simulink model "chydrbf_bruite_s"  (R2017b)
settings: Solver=ode45  StartTime=0.0  StopTime=50  MaxStep=1  MinStep=0.0001  RelTol=1e-8  AbsTol=1e-8  EnableMultiTasking=on
values from neighbouring files (symbols this model uses):
  F = [1 4.73333333333 7.10666666667 8.97333333333 2.88 0.266666666667]    [datahydr_pprTf5.mat]    (also in ppfil.m = real(poly(diag(r))))
  kw = 0.5    [datahydr_pprTf5.mat]    (also in initchydr_yuwch.m)
  R = []    [bezout.m]    (also in datahydr_pprTf5.mat = [1.68 7.4 9.48 11.84 0.8])
  S = []    [bezout.m]    (also in datahydr_pprTf5.mat = [1 4.4 8.64 8.4 5.76 0])
  T = [3 14.2 21.32 26.92 8.64 0.8]    [datahydr_pprTf5.mat]
  Ta = 10    [datahydr_pprTf5.mat]    (also in initchydr_yuwch.m)
  TI = 0.3    [datahydr_pprTf5.mat]    (also in initchydr_yuwch.m)
  Tw = 1    [datahydr_pprTf5.mat]    (also in initchydr_yuwch.m)
settings Model: Creator=pchevrel  LastModifiedBy=pchevrel
settings DataIOCC: LimitDataPoints=on  SaveFormat=Array  SignalLoggingSaveFormat=ModelDataLogs  SaveOutput=off  SaveTime=off  SignalLoggingName=sigsOut
settings OptimizationCC: ExpressionDepthLimit=2147483647  InitFltsAndDblsToZero=on  LifeSpan=inf
settings DebuggingCC: SaveWithParameterizedLinksMsg=none  UnderspecifiedInitializationDetection=Classic  MergeDetectMultiDrivingBlocksExec=none  SignalResolutionControl=TryResolveAllWithWarning  MultiTaskDSMMsg=warning  MultiTaskCondExecSysMsg=none  FcnCallInpInsideContextMsg=warning  StateNameClashWarn=warning  StrictBusMsg=None  SFUnexpectedBacktrackingDiag=warning  SFNoUnconditionalDefaultTransitionDiag=warning  SFExecutionAtInitializationDiag=none
settings HardwareCC: ProdBitPerPointer=32  ProdBitPerSizeT=32  ProdBitPerPtrDiffT=32  ProdLargestAtomicFloat=None  ProdIntDivRoundTo=Undefined  ProdEndianess=Unspecified  ProdWordSize=32  ProdHWDeviceType=32-bit Generic  TargetUnknown=on
settings ModelReferenceCC: PropagateSignalLabelsOutOfModel=off
settings CodeAppCC: StateflowObjectComments=on
settings GRTTargetCC: TargetFcnLib=ansi_tfl_tmw.mat  TargetLangStandard=C89/C90 (ANSI)  CombineOutputUpdateFcns=off  GRTInterface=on
settings ConfigComp: CovMetricSettings=dw  CovHtmlReporting=on  CovSaveCumulativeToWorkspaceVar=on  CovSaveSingleToWorkspaceVar=on  CovExternalEMLEnable=off

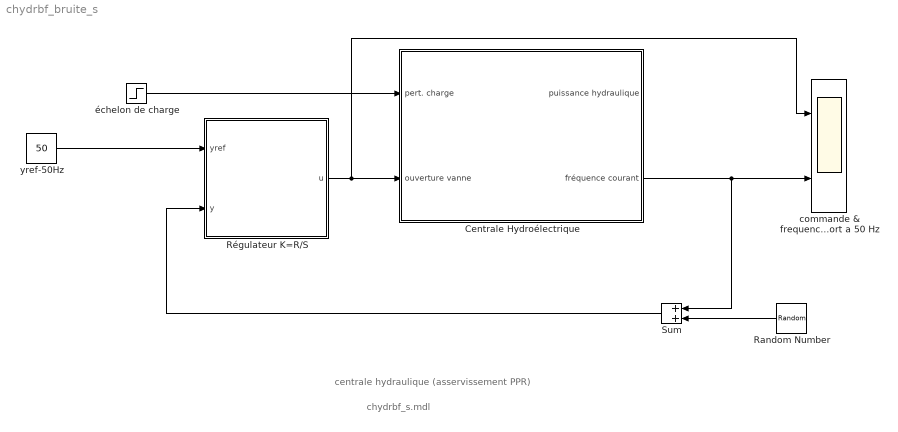
== system chydrbf_bruite_s ==
  note: chydrbf_s.mdl
  note: centrale hydraulique (asservissement PPR)
  Centrale Hydroélectrique : Subsystem
  Random Number : RandomNumber  Variance=5  SampleTime=0
  Régulateur K=R/S : Subsystem
  Sum : Sum  SaturateOnIntegerOverflow=on  InputSameDT=on  OutDataTypeStr=Inherit: Same as first input
  commande & frequence en relatif par rapport a 50 Hz : Scope  NumInputPorts=2
  yref-50Hz : Constant  Value=50
  échelon de charge : Step  Time=20  After=10  SampleTime=0
  wires:
  Centrale Hydroélectrique/2(fréquence courant) -> commande & frequence en relatif par rapport a 50 Hz/2, Sum/1
  Régulateur K=R/S/1(u) -> Centrale Hydroélectrique/2(ouverture vanne), commande & frequence en relatif par rapport a 50 Hz/1
  yref-50Hz/1 -> Régulateur K=R/S/1(yref)
  échelon de charge/1 -> Centrale Hydroélectrique/1(pert. charge)
  Sum/1 -> Régulateur K=R/S/2(y)
  Random Number/1 -> Sum/2

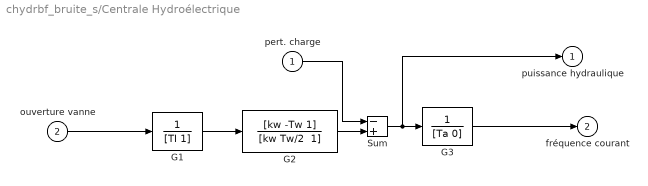
== system chydrbf_bruite_s/Centrale Hydroélectrique ==
  pert. charge : Inport
  ouverture vanne : Inport  Port=2
  G1 : TransferFcn  Denominator=[TI 1]
  G2 : TransferFcn  Numerator=[kw -Tw 1]  Denominator="[kw Tw/2  1]"
  G3 : TransferFcn  Denominator=[Ta 0]
  Sum : Sum  Inputs=-+  SaturateOnIntegerOverflow=on  InputSameDT=on  OutDataTypeStr=Inherit: Same as first input
  puissance hydraulique : Outport
  fréquence courant : Outport  Port=2
  wires:
  G2/1 -> Sum/2
  Sum/1 -> G3/1, puissance hydraulique/1
  G3/1 -> fréquence courant/1
  G1/1 -> G2/1
  pert. charge/1 -> Sum/1
  ouverture vanne/1 -> G1/1

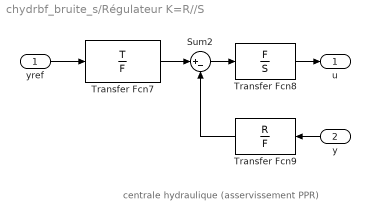
== system chydrbf_bruite_s/Régulateur K=R//S ==
  note: centrale hydraulique (asservissement PPR)
  yref : Inport
  y : Inport  Port=2
  Sum2 : Sum  Inputs=|+-  SaturateOnIntegerOverflow=on  InputSameDT=on  OutDataTypeStr=Inherit: Same as first input
  Transfer Fcn7 : TransferFcn  Numerator=T  Denominator=F
  Transfer Fcn8 : TransferFcn  Numerator=F  Denominator=S
  Transfer Fcn9 : TransferFcn  Numerator=R  Denominator=F
  u : Outport
  wires:
  Sum2/1 -> Transfer Fcn8/1
  Transfer Fcn7/1 -> Sum2/1
  Transfer Fcn9/1 -> Sum2/2
  yref/1 -> Transfer Fcn7/1
  Transfer Fcn8/1 -> u/1
  y/1 -> Transfer Fcn9/1
